simulink model "Formation_FMS1"  (R2022b)
settings: Solver=VariableStepAuto  StartTime=0.0  StopTime=10.0  RelTol=1e-3
values from neighbouring files (symbols this model uses):
  FMS_PARAM = Simulink.Parameter(FMS_PARAM_VALUE)    [fms_model_init.m]
undefined symbols (not defined in the file or in its folder): ax_cmd, ay_cmd, CONTROL_CONST, CONTROL_PARAM, CTRL_PARAM, DiscIntNeverNeededParam, FORMATION_PARAM, PilotMode, vh_cmd
libraries: FC_Lib x32, simulink x12
(part 2 of 2)

== system Formation_FMS1/FMS Commander/Commander/Mission/Mission_SubSystem/Position Command/L1 Control/L1_Core ==
  p_vehicle : Inport
  L1_WP : Inport  Port=2
  L1 : Inport  Port=3
  Vg : Inport  Port=4
  L1_Lateral_Acceleration : Subsystem
  Subtract : Sum  Inputs=+-
  ay_cmd_mPs2 : Outport  VectorParamsAs1DForOutWhenUnconnected=off
  wires:
  L1_WP/1 -> Subtract/1
  p_vehicle/1 -> Subtract/2
  L1/1 -> L1_Lateral_Acceleration/1(L1)
  Vg/1 -> L1_Lateral_Acceleration/2(Vg)
  Subtract/1 -> L1_Lateral_Acceleration/3(l1_path)
  L1_Lateral_Acceleration/1(l1_a_cmd) -> ay_cmd_mPs2/1

== system Formation_FMS1/FMS Commander/Commander/FormMission/FormMission_SubSystem/Position Command/L1 Control/L1_Core/L1_Lateral_Acceleration ==
  L1 : Inport
  Vg : Inport  Port=2
  l1_path : Inport  Port=3
  Divide : Product  Inputs=*/
  Gain : Gain  Gain=2
  Included Angle : Subsystem
  Multiply1 : Product
  Saturation : Saturate  UpperLimit=pi/2  LowerLimit=-pi/2
  Sin : Trigonometry
  Square : Math  Operator=square  SignedPower=on
  Vector Modulus : FC_Lib/Math/Vector Modulus
      settings: SourceProductName=Flight Control Toolbox
  Vector Normalize : FC_Lib/Math/Vector Normalize
      settings: SourceProductName=Flight Control Toolbox
  Vector Normalize1 : FC_Lib/Math/Vector Normalize
      settings: SourceProductName=Flight Control Toolbox
  l1_a_cmd : Outport  VectorParamsAs1DForOutWhenUnconnected=off
  wires:
  Vector Normalize/1 -> Included Angle/1(vec1)
  Included Angle/1(angle_rad) -> Saturation/1  "L1_alpha"
  Multiply1/1 -> Divide/1
  Divide/1 -> l1_a_cmd/1  "l1_a_cmd"
  Vector Normalize1/1 -> Included Angle/2(vec2)
  Sin/1 -> Multiply1/1  "sin_alpha"
  l1_path/1 -> Vector Normalize1/1
  Saturation/1 -> Sin/1
  Vg/1 -> Vector Normalize/1, Vector Modulus/1
  Square/1 -> Gain/1
  Gain/1 -> Multiply1/2
  L1/1 -> Divide/2
  Vector Modulus/1 -> Square/1

== system Formation_FMS1/FMS Commander/Commander/Mission/Mission_SubSystem/Position Command/L1 Control/L1_Core/L1_Lateral_Acceleration ==
  L1 : Inport
  Vg : Inport  Port=2
  l1_path : Inport  Port=3
  Divide : Product  Inputs=*/
  Gain : Gain  Gain=2
  Included Angle : Subsystem
  Multiply1 : Product
  Saturation : Saturate  UpperLimit=pi/2  LowerLimit=-pi/2
  Sin : Trigonometry
  Square : Math  Operator=square  SignedPower=on
  Vector Modulus : FC_Lib/Math/Vector Modulus
      settings: SourceProductName=Flight Control Toolbox
  Vector Normalize : FC_Lib/Math/Vector Normalize
      settings: SourceProductName=Flight Control Toolbox
  Vector Normalize1 : FC_Lib/Math/Vector Normalize
      settings: SourceProductName=Flight Control Toolbox
  l1_a_cmd : Outport  VectorParamsAs1DForOutWhenUnconnected=off
  wires:
  Vector Normalize/1 -> Included Angle/1(vec1)
  Included Angle/1(angle_rad) -> Saturation/1  "L1_alpha"
  Multiply1/1 -> Divide/1
  Divide/1 -> l1_a_cmd/1  "l1_a_cmd"
  Vector Normalize1/1 -> Included Angle/2(vec2)
  Sin/1 -> Multiply1/1  "sin_alpha"
  l1_path/1 -> Vector Normalize1/1
  Saturation/1 -> Sin/1
  Vg/1 -> Vector Normalize/1, Vector Modulus/1
  Square/1 -> Gain/1
  Gain/1 -> Multiply1/2
  L1/1 -> Divide/2
  Vector Modulus/1 -> Square/1

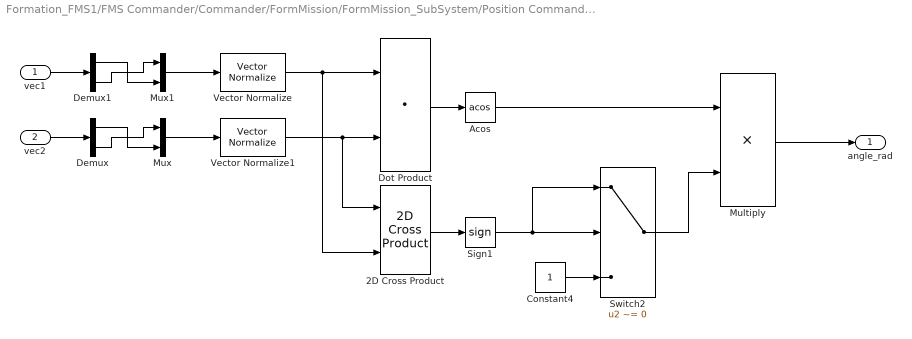
== system Formation_FMS1/FMS Commander/Commander/FormMission/FormMission_SubSystem/Position Command/L1 Control/L1_Core/L1_Lateral_Acceleration/Included Angle ==
  vec1 : Inport
  vec2 : Inport  Port=2
  2D Cross Product : FC_Lib/Math/2D Cross Product
      settings: SourceProductName=Flight Control Toolbox
  Acos : Trigonometry  Operator=acos
  Constant4 : Constant  OutDataTypeStr=single
  Demux : Demux  Outputs=2
  Demux1 : Demux  Outputs=2
  Dot Product : DotProduct  OutDataTypeStr=Inherit: Inherit via internal rule
  Multiply : Product
  Mux : Mux  Inputs=2
  Mux1 : Mux  Inputs=2
  Sign1 : Signum
  Switch2 : Switch  Criteria=u2 ~= 0  SaturateOnIntegerOverflow=off  InputSameDT=off
  Vector Normalize : FC_Lib/Math/Vector Normalize
      settings: SourceProductName=Flight Control Toolbox
  Vector Normalize1 : FC_Lib/Math/Vector Normalize
      settings: SourceProductName=Flight Control Toolbox
  angle_rad : Outport  VectorParamsAs1DForOutWhenUnconnected=off
  wires:
  Switch2/1 -> Multiply/2
  Acos/1 -> Multiply/1
  Mux/1 -> Vector Normalize1/1
  vec2/1 -> Demux/1
  Constant4/1 -> Switch2/3
  Demux/1 -> Mux/2
  vec1/1 -> Demux1/1
  Multiply/1 -> angle_rad/1
  2D Cross Product/1 -> Sign1/1
  Vector Normalize/1 -> 2D Cross Product/2, Dot Product/1
  Demux/2 -> Mux/1
  Vector Normalize1/1 -> 2D Cross Product/1, Dot Product/2
  Sign1/1 -> Switch2/2, Switch2/1
  Demux1/2 -> Mux1/1
  Mux1/1 -> Vector Normalize/1
  Demux1/1 -> Mux1/2
  Dot Product/1 -> Acos/1

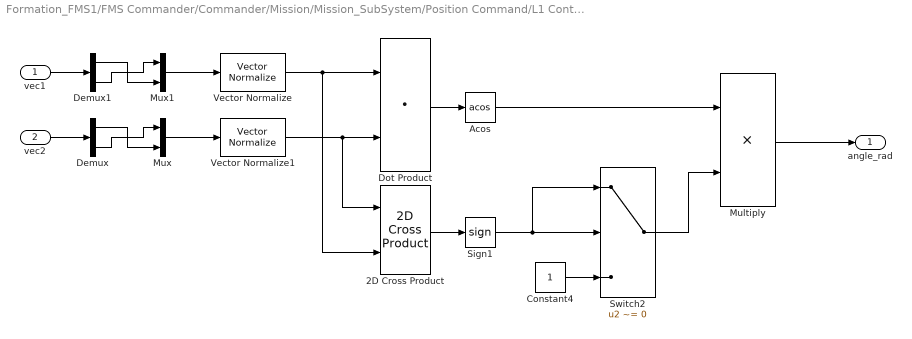
== system Formation_FMS1/FMS Commander/Commander/Mission/Mission_SubSystem/Position Command/L1 Control/L1_Core/L1_Lateral_Acceleration/Included Angle ==
  vec1 : Inport
  vec2 : Inport  Port=2
  2D Cross Product : FC_Lib/Math/2D Cross Product
      settings: SourceProductName=Flight Control Toolbox
  Acos : Trigonometry  Operator=acos
  Constant4 : Constant  OutDataTypeStr=single
  Demux : Demux  Outputs=2
  Demux1 : Demux  Outputs=2
  Dot Product : DotProduct  OutDataTypeStr=Inherit: Inherit via internal rule
  Multiply : Product
  Mux : Mux  Inputs=2
  Mux1 : Mux  Inputs=2
  Sign1 : Signum
  Switch2 : Switch  Criteria=u2 ~= 0  SaturateOnIntegerOverflow=off  InputSameDT=off
  Vector Normalize : FC_Lib/Math/Vector Normalize
      settings: SourceProductName=Flight Control Toolbox
  Vector Normalize1 : FC_Lib/Math/Vector Normalize
      settings: SourceProductName=Flight Control Toolbox
  angle_rad : Outport  VectorParamsAs1DForOutWhenUnconnected=off
  wires:
  Switch2/1 -> Multiply/2
  Acos/1 -> Multiply/1
  Mux/1 -> Vector Normalize1/1
  vec2/1 -> Demux/1
  Constant4/1 -> Switch2/3
  Demux/1 -> Mux/2
  vec1/1 -> Demux1/1
  Multiply/1 -> angle_rad/1
  2D Cross Product/1 -> Sign1/1
  Vector Normalize/1 -> 2D Cross Product/2, Dot Product/1
  Demux/2 -> Mux/1
  Vector Normalize1/1 -> 2D Cross Product/1, Dot Product/2
  Sign1/1 -> Switch2/2, Switch2/1
  Demux1/2 -> Mux1/1
  Mux1/1 -> Vector Normalize/1
  Demux1/1 -> Mux1/2
  Dot Product/1 -> Acos/1

== matlab function Formation_FMS1/FMS Commander/Commander/Default/Loiter_Control/L1 Reference WP/OutRegionRegWP ==
  data: P0 input; P output; P_Vehicle input; R input; L1 input; n input
% Find the reference waypoint when vehicle has no intersection with loicter circle.
%
% There are two region defined:
%   Region 1: The vehicle is outside of loiter circle
%   Region 2: The else situation
%
function P = OutRegionRefWP(P0, P_Vehicle, R, L1, n)

if sum((P_Vehicle-P0).^2) > R^2
    % outside of loiter circle, we just select P0 as P
    P = P0;
else
    % inside of loiter circle, we just let vehicle keep current direction
    P = P_Vehicle + n*L1;
end

== matlab function Formation_FMS1/FMS Commander/Commander/Default/Loiter_Control/L1 Reference WP/SearchL1RefWP ==
  data: P_0 input; P output; P_Vehicle input; R input; L1 input; n output
% Find reference waypoint (L1RefWP) on the loiter circle with origin at 
% P_0 and radius of R
%
% The idea is to calculate the intersection point of 2 circles (P_0:R and
% P_Vehicle:L1).
% Refer to: Knut Andreas Lie's Unstructured PEBI-grids Adapting to Geological Features in Subsurface Reservoirs
%
% Input:
%   P_0: loiter circle origin
%   P_Vehicle: vehicle position
%   R: loiter radius
%   L1: the L1 distance
% Output:
%   P: L1 reference waypoint
%   n: number of intersection points.
function [P, n] = SearchL1RefWP(P_0, P_Vehicle, R, L1)

C0 = P_Vehicle;
R0 = L1;
C1 = P_0;
R1 = R;
P = single([0;0]);

if C0(1)==C1(1) && C0(2)==C1(2) && R==L1
   % we have 2 same circle
   n = 0;
   return;
end

d = sqrt(sum((C1-C0).^2));
a = (d^2 + R0^2 - R1^2) / (2*d);

% n1 is perpendicular to n0
n0 = (C1-C0)/d;
n1 = [0 -1; 1 0] * n0;

if a^2 > R0^2
    % no intersection
    n = 0;
elseif a^2 == R0^2
    % only 1 intersection
    n = 1;
    P = C0 + a*n0;
else
    % 2 intersection
    n = 2;
    % we always choose the point with clockwise direction,
    % if wants anti-clockwise direction, choose h = -sqrt(R0^2 - a^2)
    h = sqrt(R0^2 - a^2);
    P = C0 + a*n0 + h*n1; 
end

== stateflow chart Formation_FMS1/FMS State Machine ==
  state Vehicle
    state Formation
      state FormAssemble
        en:
        if is_leader
        Other_Mission_Data = dubinsPath(Other_INS_Out);
        end
        state Other_Mission_Data = dubinsPath(Other_INS_Out) [function]
        state NextWP
          en:
          state = VehicleState.FormAssemble;
        state Waypoint
          en:
          % set current waypoint to previous setpoint waypoint
          Cmd_In.cur_waypoint = Cmd_In.sp_waypoint;
          % Geodetic coordinates (latitude, longitude, and altitude), specified as an m-by-3 array in [degrees degrees meters]
          % Altitude add home(3) here because the altitude when takeoff could be non-zero
          % lla = [double(Mission_Data.x(wp_index))*1e-7, double(Mission_Data.y(wp_index))*1e-7, double(-(Mission_Data.z(wp_index) + home(3)))];
          % target waypoint
          Cmd_In.sp_waypoint = [Mission_Data.x(wp_index); Mission_Data.y(wp_index); Mission_Data.z(wp_index)];%LLA2FLAT(lla, llo, 0, 0);
        state WaitForUpdate
          en:
          state = VehicleState.None;
        (junction 206) -> (junction 197) : {wp_index = wp_index + 1;}
        (junction 197) -> Vehicle.Formation.FormAssemble.NextWP
        (junction 215) -> (junction 206)
        WaitForUpdate -> Vehicle.Formation.FormAssemble.NextWP : [hasChanged(Mission_Data.timestamp)]{wp_index=1;}
        (default) -> WaitForUpdate
        Vehicle.Formation.FormAssemble.Waypoint -> (junction 215) : [norm([INS_Out.x_R;INS_Out.y_R]-Cmd_In.sp_waypoint(1:2)) <= accept_radius]
        Vehicle.Formation.FormAssemble.NextWP -> Vehicle.Formation.FormAssemble.Waypoint [order 1] : [wp_index <= Mission_Data.valid_items]
      state FormMission
        en:
        % Reference location of latitude and longitude, specified as an m-by-2 array, in degrees
        % llo = [INS_Out.lat_0, INS_Out.lon_0] * (180/pi);
        % Upon enter Mission mode, set current position as setpoint waypoint
        Cmd_In.sp_waypoint = [INS_Out.x_R; INS_Out.y_R; INS_Out.h_R];
        state = VehicleState.FormMission;
        state NextWP
        state Waypoint
          en:
          % set current waypoint to previous setpoint waypoint
          Cmd_In.cur_waypoint = Cmd_In.sp_waypoint;
          % Geodetic coordinates (latitude, longitude, and altitude), specified as an m-by-3 array in [degrees degrees meters]
          % Altitude add home(3) here because the altitude when takeoff could be non-zero
          % lla = [double(Mission_Data.x(wp_index))*1e-7, double(Mission_Data.y(wp_index))*1e-7, double(-(Mission_Data.z(wp_index) + home(3)))];
          % target waypoint
          Cmd_In.sp_waypoint = [Mission_Data.x(wp_index); Mission_Data.y(wp_index); Mission_Data.z(wp_index)];%LLA2FLAT(lla, llo, 0, 0);
          Cmd_In.l1_enable = true;
        state Follower
          en:
          Cmd_In.l1_enable = false;
        state Forward
          en:
          Cmd_In.l1_enable = false;
        (junction 83) -> (junction 82) : {wp_index = wp_index + 1;}
        (junction 82) -> Vehicle.Formation.FormMission.NextWP
        (junction 84) -> (junction 83)
        (default) -> Vehicle.Formation.FormMission.NextWP
        Vehicle.Formation.FormMission.NextWP -> Vehicle.Formation.FormMission.Waypoint [order 2] : [wp_index <= Mission_Data.valid_items]
        Vehicle.Formation.FormMission.Waypoint -> (junction 84) : [norm([INS_Out.x_R;INS_Out.y_R]-Cmd_In.sp_waypoint(1:2)) <= accept_radius]
        FormMission -> Vehicle.Formation.FormMission.NextWP [order 1] : [hasChanged(Mission_Data.timestamp)]{wp_index=1;}
        Vehicle.Formation.FormMission.NextWP -> Follower [order 1] : [~is_leader]
        Vehicle.Formation.FormMission.NextWP -> Forward [order 3]
      state FormDisband
        en:
        state=VehicleState.FormDisband;
      state InvalidMode
      Vehicle.Formation.FormAssemble.NextWP -> FormMission [order 2]
      (default) -> (junction 97)
      (junction 97) -> FormAssemble [order 1] : [mode==PilotMode.FormAssemble]
      (junction 97) -> InvalidMode [order 2]
      FormMission -> FormDisband [order 1] : [mode==PilotMode.FormDisband]
    state Mission
      en:
      % Reference location of latitude and longitude, specified as an m-by-2 array, in degrees
      % llo = [INS_Out.lat_0, INS_Out.lon_0] * (180/pi);
      % Upon enter Mission mode, set current position as setpoint waypoint
      Cmd_In.sp_waypoint = [INS_Out.x_R; INS_Out.y_R; INS_Out.h_R];
      state NextWP
        en:
        state = VehicleState.None;
      state Waypoint
        en:
        % set current waypoint to previous setpoint waypoint
        Cmd_In.cur_waypoint = Cmd_In.sp_waypoint;
        % Geodetic coordinates (latitude, longitude, and altitude), specified as an m-by-3 array in [degrees degrees meters]
        % Altitude add home(3) here because the altitude when takeoff could be non-zero
        % lla = [double(Mission_Data.x(wp_index))*1e-7, double(Mission_Data.y(wp_index))*1e-7, double(-(Mission_Data.z(wp_index) + home(3)))];
        % target waypoint
        Cmd_In.sp_waypoint = [Mission_Data.x(wp_index); Mission_Data.y(wp_index); Mission_Data.z(wp_index)];%LLA2FLAT(lla, llo, 0, 0);
        state = VehicleState.Mission;
      state Loiter
        en:
        Cmd_In.cur_waypoint = Cmd_In.sp_waypoint;
        state = VehicleState.Hold;
      (junction 6) -> (junction 5) : {wp_index = wp_index + 1;}
      (junction 9) -> (junction 6)
      (junction 5) -> Vehicle.Mission.NextWP
      (default) -> Vehicle.Mission.NextWP
      Vehicle.Mission.NextWP -> Vehicle.Mission.Waypoint [order 1] : [wp_index <= Mission_Data.valid_items]
      Vehicle.Mission.Waypoint -> (junction 9) : [norm([INS_Out.x_R;INS_Out.y_R]-Cmd_In.sp_waypoint(1:2)) <= accept_radius]
      Mission -> Vehicle.Mission.NextWP : [hasChanged(Mission_Data.timestamp)]{wp_index=1;}
      Vehicle.Mission.NextWP -> Loiter [order 2] : [wp_index > Mission_Data.valid_items]
    state Standby
      en:
      Cmd_In.cur_waypoint = [INS_Out.x_R; INS_Out.y_R; INS_Out.h_R];
      state = VehicleState.Hold;
    Vehicle -> (junction 62) : [hasChanged(mode) && mode ~= PilotMode.None]
    (default) -> (junction 62)
    (junction 62) -> Formation [order 1] : [any(mode==[PilotMode.FormAssemble,PilotMode.FormDisband])]
    (junction 62) -> (junction 67) [order 2]
    (junction 67) -> Mission [order 1] : [mode==PilotMode.Mission]{wp_index=1;
        | Cmd_In.cur_waypoint = [INS_Out.x_R; INS_Out.y_R; INS_Out.h_R];
        | }
    (junction 67) -> (junction 78) [order 2]
    InvalidMode -> Standby
    (junction 78) -> Standby
  data: Other_INS_Out function_input Bus: Other_INS_Out_Bus size=1; Other_Mission_Data function_output Bus: Other_Mission_Data_Bus size=1; INS_Out input Bus: INS_Out_Bus; Other_INS_Out input; mode input Enum: PilotMode; Mission_Data input Bus: Mission_Data_Bus; is_leader input; state output Enum: VehicleState; Cmd_In output Bus: Commander_In_Bus; wp_index output uint16; accept_radius input; Other_Mission_Data output Bus: Other_Mission_Data_Bus

== matlab function Formation_FMS1/FMS Commander/Commander/FormMission/FormMission_SubSystem/Position Command/L1 Control/L1 Reference WP/NearbyRefWP ==
  data: P output; P2 input; d output; P3 input; L1 input
% Find the reference waypoint when vehicle (P3) is close to target (P2)
%
% If the vehicle is close to target (distance(P2,P3) < L1), select P2 as
% reference waypoint and return the distance, otherwise return -1.
function [P,d] = NearbyRefWP(P2, P3, L1)

P3P2 = P2 - P3;
dis = sqrt(sum(P3P2.^2));

if dis <= L1
    d = dis;
    % select P2 as reference WP
    P = P2;
else
    d = single(-1);
    % unset WP
    P = single([0; 0]);
end

== matlab function Formation_FMS1/FMS Commander/Commander/Hold/Loiter_Control/L1 Reference WP/OutRegionRegWP ==
  data: P0 input; P output; P_Vehicle input; R input; L1 input; n input
% Find the reference waypoint when vehicle has no intersection with loicter circle.
%
% There are two region defined:
%   Region 1: The vehicle is outside of loiter circle
%   Region 2: The else situation
%
function P = OutRegionRefWP(P0, P_Vehicle, R, L1, n)

if sum((P_Vehicle-P0).^2) > R^2
    % outside of loiter circle, we just select P0 as P
    P = P0;
else
    % inside of loiter circle, we just let vehicle keep current direction
    P = P_Vehicle + n*L1;
end

== matlab function Formation_FMS1/FMS Commander/Commander/Mission/Mission_SubSystem/Position Command/L1 Control/L1 Reference WP/NearbyRefWP ==
  data: P output; P2 input; d output; P3 input; L1 input
% Find the reference waypoint when vehicle (P3) is close to target (P2)
%
% If the vehicle is close to target (distance(P2,P3) < L1), select P2 as
% reference waypoint and return the distance, otherwise return -1.
function [P,d] = NearbyRefWP(P2, P3, L1)

P3P2 = P2 - P3;
dis = sqrt(sum(P3P2.^2));

if dis <= L1
    d = dis;
    % select P2 as reference WP
    P = P2;
else
    d = single(-1);
    % unset WP
    P = single([0; 0]);
end

== matlab function Formation_FMS1/FMS Commander/Commander/FormMission/FormMission_SubSystem/Position Command/L1 Control/L1 Reference WP/OutRegionRegWP ==
  data: P1 input; P output; P2 input; P3 input
% Find the reference waypoint when vehicle is out of L1 region near P1P2.
%
% There are three region defined:
%   Region 1: The project point of P3 is lied on left side of P1P2
%   Region 2: The project point of P3 is lied on right side of P1P2
%   Region 3: The project point of P3 is lied on the segment line 
%
%   For the case of region 3, we select the project point as the reference
%   wayspoint. For the case of region 1, we choose P1 as reference waypoint
%   and similarly for the case of region 2, we choose P3 as reference
%   waypoint.
function P = OutRegionRefWP(P1, P2, P3)
% segment line P1P2
P1P2 = P2 - P1;
% segment line P1P3
P1P3 = P3 - P1;

% Define C as the P3 project point on line P1P2.
% Hence, P1C = dot(P1P3, P1P2)/|P1P2| * (P1P2/|P1P2|) = u * P1P2
% where u = dot(P1P3, P1P2) / |P1P2|^2.
u = dot(P1P3, P1P2) / sum(P1P2.^2);

if u <= 0
    % region 1
    P = P1;
elseif u >= 1
    % region 2
    P = P2;
else
    % region 3. C = P1C + P1
    % P = u * P1P2 + P1;
    
    C = u * P1P2 + P1;
    % tan(pi/6) = 0.5774
    u = sqrt(sum((C-P3).^2))*single(0.5774)/sqrt(sum(P1P2.^2)) + u;
    if u > 1
        u = single(1);
    end
    P = u * P1P2 + P1;
end

== matlab function Formation_FMS1/FMS Commander/Commander/Mission/Mission_SubSystem/Position Command/L1 Control/L1 Reference WP/OutRegionRegWP ==
  data: P1 input; P output; P2 input; P3 input
% Find the reference waypoint when vehicle is out of L1 region near P1P2.
%
% There are three region defined:
%   Region 1: The project point of P3 is lied on left side of P1P2
%   Region 2: The project point of P3 is lied on right side of P1P2
%   Region 3: The project point of P3 is lied on the segment line 
%
%   For the case of region 3, we select the project point as the reference
%   wayspoint. For the case of region 1, we choose P1 as reference waypoint
%   and similarly for the case of region 2, we choose P3 as reference
%   waypoint.
function P = OutRegionRefWP(P1, P2, P3)
% segment line P1P2
P1P2 = P2 - P1;
% segment line P1P3
P1P3 = P3 - P1;

% Define C as the P3 project point on line P1P2.
% Hence, P1C = dot(P1P3, P1P2)/|P1P2| * (P1P2/|P1P2|) = u * P1P2
% where u = dot(P1P3, P1P2) / |P1P2|^2.
u = dot(P1P3, P1P2) / sum(P1P2.^2);

if u <= 0
    % region 1
    P = P1;
elseif u >= 1
    % region 2
    P = P2;
else
    % region 3. C = P1C + P1
    % P = u * P1P2 + P1;
    
    C = u * P1P2 + P1;
    % tan(pi/6) = 0.5774
    u = sqrt(sum((C-P3).^2))*single(0.5774)/sqrt(sum(P1P2.^2)) + u;
    if u > 1
        u = single(1);
    end
    P = u * P1P2 + P1;
end

== matlab function Formation_FMS1/FMS Commander/Commander/Mission/Mission_SubSystem/Position Command/L1 Control/L1 Reference WP/SearchL1RefWP ==
  data: P1 input; P output; P2 input; P3 input; L1 input; u output
% Find reference waypoint (L1RefWP) on the line segment P1P2 which has 
% L1 distance from vehicle position (P3).
%
% The idea is to calculate the intersection point of a circle with L1 radius
% with the line segment P1P2.
%
% Define P = P1 + u * (P2 - P1), where P is the intersection point.
% Goal is calculating the u, where the valid u is between [0, 1].
%
% Input:
%   P1: start point of segment line
%   P2: start point of segment line
%   P3: circle center point, also is known as the vehicle position
%   L1: the L1 distance
% Output:
%   P: L1 reference waypoint
%   u: scale factor (valid between 0 and 1), -1 means no intersection.
function [P, u] = SearchL1RefWP(P1, P2, P3, L1)

% P1 = (x1, y1), P2 = (x2, y2), P3 = (x3, y3)
x1 = P1(1);
y1 = P1(2);
x2 = P2(1);
y2 = P2(2);
x3 = P3(1);
y3 = P3(2);

% The P is on circle and line segment, which yields:
A = (x2 - x1)^2 + (y2 - y1)^2;
B = 2 * ((x2 - x1)*(x1 - x3) + (y2 - y1)*(y1 - y3));
C = x3^2 + y3^2 + x1^2 + y1^2 - 2*(x3*x1 + y3*y1) - L1^2;
% Check root existence confition if B^2 - 4*A*C >= 0
D = B^2 - 4*A*C;
u = single(-1);
P = single([0 0]);

if D > 0
    % D>0 means we have 2 difference roots, % root is valid only if u is in range of [0, 1]
    u1 = (-B + sqrt(D)) / (2*A);
    u2 = (-B - sqrt(D)) / (2*A);
    
    if (u1>=0 && u1<=1) && (u2>=0 && u2<=1)
        % have 2 valid roots, select the one which is closer to P2 (target point)
        if u1 > u2
            u = u1; 
        else
            u = u2;
        end
    elseif (u1>=0 && u1<=1)
        % only 1 root valid, select it
        u = u1;
    elseif (u2>=0 && u2<=1)
        % only 1 root valid, select it
        u = u2;
    else
        % no valid root, which means no intersection point founded.
        return;
    end
elseif D == 0
    % D=0 means only 1 single root
    u1 = -B / (2*A);
    if (u1>=0 && u1<=1)
        % valid root, select it
        u = u1;
    else
        % no valid root, which means no intersection point founded.
        return;
    end
else
    % no valid root, which means no intersection point founded.
    return;
end

% calculate the L1 reference waypoint (P) coordinate
P(1) = x1 + u*(x2 - x1);
P(2) = y1 + u*(y2 - y1);

== matlab function Formation_FMS1/FMS Commander/Commander/FormMission/FormMission_SubSystem/Position Command/L1 Control/L1 Reference WP/SearchL1RefWP ==
  data: P1 input; P output; P2 input; P3 input; L1 input; u output
% Find reference waypoint (L1RefWP) on the line segment P1P2 which has 
% L1 distance from vehicle position (P3).
%
% The idea is to calculate the intersection point of a circle with L1 radius
% with the line segment P1P2.
%
% Define P = P1 + u * (P2 - P1), where P is the intersection point.
% Goal is calculating the u, where the valid u is between [0, 1].
%
% Input:
%   P1: start point of segment line
%   P2: start point of segment line
%   P3: circle center point, also is known as the vehicle position
%   L1: the L1 distance
% Output:
%   P: L1 reference waypoint
%   u: scale factor (valid between 0 and 1), -1 means no intersection.
function [P, u] = SearchL1RefWP(P1, P2, P3, L1)

% P1 = (x1, y1), P2 = (x2, y2), P3 = (x3, y3)
x1 = P1(1);
y1 = P1(2);
x2 = P2(1);
y2 = P2(2);
x3 = P3(1);
y3 = P3(2);

% The P is on circle and line segment, which yields:
A = (x2 - x1)^2 + (y2 - y1)^2;
B = 2 * ((x2 - x1)*(x1 - x3) + (y2 - y1)*(y1 - y3));
C = x3^2 + y3^2 + x1^2 + y1^2 - 2*(x3*x1 + y3*y1) - L1^2;
% Check root existence confition if B^2 - 4*A*C >= 0
D = B^2 - 4*A*C;
u = single(-1);
P = single([0 0]);

if D > 0
    % D>0 means we have 2 difference roots, % root is valid only if u is in range of [0, 1]
    u1 = (-B + sqrt(D)) / (2*A);
    u2 = (-B - sqrt(D)) / (2*A);
    
    if (u1>=0 && u1<=1) && (u2>=0 && u2<=1)
        % have 2 valid roots, select the one which is closer to P2 (target point)
        if u1 > u2
            u = u1; 
        else
            u = u2;
        end
    elseif (u1>=0 && u1<=1)
        % only 1 root valid, select it
        u = u1;
    elseif (u2>=0 && u2<=1)
        % only 1 root valid, select it
        u = u2;
    else
        % no valid root, which means no intersection point founded.
        return;
    end
elseif D == 0
    % D=0 means only 1 single root
    u1 = -B / (2*A);
    if (u1>=0 && u1<=1)
        % valid root, select it
        u = u1;
    else
        % no valid root, which means no intersection point founded.
        return;
    end
else
    % no valid root, which means no intersection point founded.
    return;
end

% calculate the L1 reference waypoint (P) coordinate
P(1) = x1 + u*(x2 - x1);
P(2) = y1 + u*(y2 - y1);

== matlab function Formation_FMS1/FMS State Machine/Vehicle.Formation.FormAssemble.dubinsPath/MATLAB Function ==
  data: ins input Bus: Other_INS_Out_Bus; mission output Bus: Other_Mission_Data_Bus; form_points parameter
function mission = fcn(ins, form_points)
pose = double([ins.x_R ins.y_R atan2(ins.vn, ins.ve)]); % 3 x 3
result = MutiDubins(pose, form_points, [25 25 25], 40);
persistent tick;
if isempty(tick)
    tick = uint32(0);
end
tick = tick + 1;
mission.timestamp = tick;
mission.valid_items = uint8([5 5 5]');
mission.x = zeros([3, 8], 'single');
mission.y = zeros([3, 8], 'single');
mission.z = zeros([3, 8], 'single');
for i = 1 : size(result, 3)
    mission.x(i, 1:5) = result(:, 1, i);
    mission.y(i, 1:5) = result(:, 2, i);
    mission.z(i, 1:5) = ins.h_R(i);
end

== matlab function Formation_FMS1/FMS Commander/Commander/Hold/Loiter_Control/L1 Reference WP/SearchL1RefWP ==
  data: P_0 input; P output; P_Vehicle input; R input; L1 input; n output
% Find reference waypoint (L1RefWP) on the loiter circle with origin at 
% P_0 and radius of R
%
% The idea is to calculate the intersection point of 2 circles (P_0:R and
% P_Vehicle:L1).
% Refer to: Knut Andreas Lie's Unstructured PEBI-grids Adapting to Geological Features in Subsurface Reservoirs
%
% Input:
%   P_0: loiter circle origin
%   P_Vehicle: vehicle position
%   R: loiter radius
%   L1: the L1 distance
% Output:
%   P: L1 reference waypoint
%   n: number of intersection points.
function [P, n] = SearchL1RefWP(P_0, P_Vehicle, R, L1)

C0 = P_Vehicle;
R0 = L1;
C1 = P_0;
R1 = R;
P = single([0;0]);

if C0(1)==C1(1) && C0(2)==C1(2) && R==L1
   % we have 2 same circle
   n = 0;
   return;
end

d = sqrt(sum((C1-C0).^2));
a = (d^2 + R0^2 - R1^2) / (2*d);

% n1 is perpendicular to n0
n0 = (C1-C0)/d;
n1 = [0 -1; 1 0] * n0;

if a^2 > R0^2
    % no intersection
    n = 0;
elseif a^2 == R0^2
    % only 1 intersection
    n = 1;
    P = C0 + a*n0;
else
    % 2 intersection
    n = 2;
    % we always choose the point with clockwise direction,
    % if wants anti-clockwise direction, choose h = -sqrt(R0^2 - a^2)
    h = sqrt(R0^2 - a^2);
    P = C0 + a*n0 + h*n1; 
end
